simulink model "SystemPIDClosedLoop_motor_closed_zrate_cascade"  (Simulink 8.3)
settings: Solver=ode4  StartTime=0.0  StopTime=100  FixedStep=0.001  RelTol=1e-3
values from neighbouring files (symbols this model uses):
  controller = [12;  38; 4]    [layer_values.m]    (also in learnonline.m = in(end-10:end-8); learnonline1.m = in(end-10:end-8); learnonline_trial.m = in(end-10:end-8))
  delta = ones(1,4)    [ROC.m]    (also in learnonline1.m = in(end-42-((4+1)*12+(12+1)*12+(12+1)*1):end-43))
  nn_params = [Theta1(:) ; Theta2(:); Theta3(:); Theta1(:) ; Theta2(:); Theta3(:)]    [checkNNGradients.m]    (also in controller_ANN.m = in(17:end-3); jkhsgdk.m = ones(3999,1); layer_values.m = [Theta1(:); Theta2(:); Theta3(:); Theta4(:); Theta5(:); Thet; learnonline.m = [Thetap1(:); Thetap2(:); Thetap3(:); Thetac1(:); Thetac2(:);)
  plant = [14; 44; 4]    [layer_values.m]    (also in learnonline.m = in(end-13 :end-11); learnonline1.m = in(end-13 :end-11); learnonline_trial.m = in(end-13 :end-11))
undefined symbols (not defined in the file or in its folder): sumy
libraries: simulink x6, aerolibfltsims x1
settings Model: Creator=Rakhi  LastModifiedBy=binabakshi
settings SolverCC: PositivePriorityOrder=on
settings OptimizationCC: ExpressionDepthLimit=2147483647
settings DebuggingCC: FcnCallInpInsideContextMsg=UseLocalSettings
settings HardwareCC: TargetBitPerLong=64  TargetBitPerPointer=64  TargetLongLongMode=on  TargetIntDivRoundTo=Zero  TargetEndianess=LittleEndian  TargetWordSize=64  TargetHWDeviceType=MATLAB Host  ProdEqTarget=off
settings RTWCC: ProcessScript=grt_make_rtw_hook
settings GRTTargetCC: CombineOutputUpdateFcns=on  GRTInterface=off
settings ConfigurationSet: Description=SimMechanics 2G

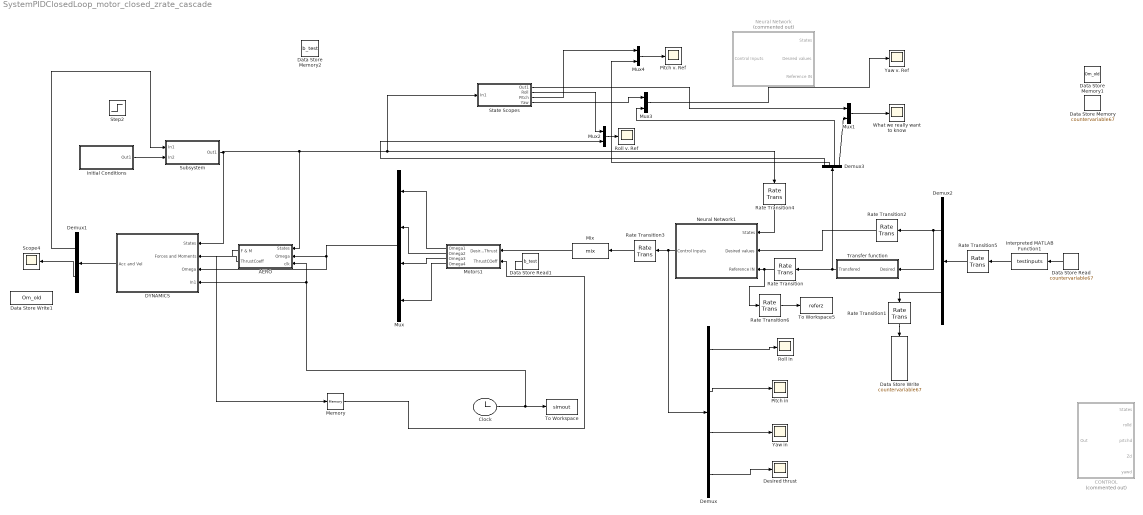
== system SystemPIDClosedLoop_motor_closed_zrate_cascade ==
  AERO : Subsystem
  CONTROL : Subsystem  Commented=on
      settings: AttributesFormatString=%<Priority>
  Clock : Clock
  DYNAMICS : Subsystem
  Data Store Memory : DataStoreMemory  DataStoreName=countervariable67
  Data Store Memory1 : DataStoreMemory  DataStoreName=Om_old  ReadBeforeWriteMsg=warning  WriteAfterWriteMsg=warning  WriteAfterReadMsg=warning
  Data Store Memory2 : DataStoreMemory  DataStoreName=b_test  ReadBeforeWriteMsg=warning  WriteAfterWriteMsg=warning  WriteAfterReadMsg=warning  InitialValue=0.000031752
  Data Store Read : DataStoreRead  DataStoreName=countervariable67  SampleTime=0.01  DataStoreElements=countervariable67
  Data Store Read1 : DataStoreRead  DataStoreName=b_test  DataStoreElements=b_test
  Data Store Write : DataStoreWrite  DataStoreName=countervariable67  DataStoreElements=countervariable67
  Data Store Write1 : DataStoreWrite  DataStoreName=Om_old  DataStoreElements=Om_old
  Demux : Demux
  Demux1 : Demux  Outputs=[12 1]
  Demux2 : Demux  Outputs=[4 1]
  Demux3 : Demux  Outputs=[1 1 1 1]
  Desired thrust : Scope
      settings: YMin=4  YMax=12  SaveName=ScopeData3
  Initial Conditions : Subsystem
  Interpreted MATLAB Function1 : MATLABFcn  MATLABFcn=testinputs  OutputDimensions=5
  Memory : Memory  X0=3.1751e-5  InheritSampleTime=on
  Mix : MATLABFcn  MATLABFcn=mix  OutputDimensions=4
  Motors1 : Subsystem
  Mux : Mux
  Mux{1..4} (4 alike) : Mux  Inputs=2
  Neural Network : Subsystem  Commented=on
  Neural Network1 : Subsystem
  Pitch in : Scope
      settings: YMin=-0.004  YMax=0.005  SaveName=ScopeData2
  Pitch v. Ref : Scope
      settings: YMin=0  YMax=0.3  SaveName=ScopeData38
  Rate Transition{,1..2,4} (4 alike) : RateTransition  OutPortSampleTime=0.01
  Rate Transition3 : RateTransition  OutPortSampleTime=0.001
  Rate Transition5 : RateTransition  OutPortSampleTime=0.001
  Rate Transition6 : RateTransition  OutPortSampleTime=0.1
  Roll in : Scope
      settings: YMin=-0.005  YMax=0.005
  Roll v. Ref : Scope
      settings: YMin=-0.2  YMax=0.5  SaveName=ScopeData35
  Scope4 : Scope
      settings: SaveName=ScopeData4
  State Scopes : Subsystem
  Subsystem : Subsystem
  To Workspace : ToWorkspace  VariableName=simout  SaveFormat=Structure  SampleTime=-1
      settings: MaxDataPoints=1
  To Workspace5 : ToWorkspace  VariableName=referz  SaveFormat=Timeseries  SampleTime=-1
      settings: MaxDataPoints=10000
  Transfer function : Subsystem
  "What we really want to know " : Scope
      settings: YMin=-3.25  YMax=0  SaveName=ScopeData32
  Yaw in : Scope
      settings: YMin=-0.45  YMax=0.5
  Yaw v. Ref : Scope
      settings: TimeRange=100  YMin=-1.5  YMax=5.5  SaveName=ScopeData37
  Step2 : Step  IOType=siggen  SampleTime=0
  wires:
  AERO/1(F & M) -> DYNAMICS/2(Forces and Moments)
  Initial Conditions/1(Out1) -> Subsystem/2(In2)
  Subsystem/1(Out1) -> DYNAMICS/1(States), AERO/1(States), Rate Transition4/1, State Scopes/1(In1)
  Demux/1 -> Roll in/1
  Demux/2 -> Pitch in/1
  Demux/4 -> Desired thrust/1
  Demux1/1 -> Subsystem/1(In1)
  DYNAMICS/1(Acc and Vel) -> Demux1/1
  Demux1/2 -> Scope4/1
  Clock/1 -> To Workspace/1, DYNAMICS/4(In1), AERO/3(clk)
  Demux/3 -> Yaw in/1
  AERO/2(ThrustCoeff) -> Memory/1
  Mix/1 -> Motors1/1(DesiredThrust)
  Data Store Read/1 -> Interpreted MATLAB Function1/1
  Mux/1 -> DYNAMICS/3(Omega), AERO/2(Omega)
  Motors1/1(Omega1) -> Mux/1
  Motors1/2(Omega2) -> Mux/2
  Motors1/3(Omega3) -> Mux/3
  Motors1/4(Omega4) -> Mux/4
  Demux2/2 -> Rate Transition1/1
  Interpreted MATLAB Function1/1 -> Rate Transition5/1
  Rate Transition1/1 -> Data Store Write/1
  Transfer function/1(Transfered) -> Rate Transition/1, Demux3/1
  Neural Network1/1(Control Inputs) -> Rate Transition3/1, Demux/1
  Demux2/1 -> Transfer function/1(Desired), Rate Transition2/1
  Rate Transition4/1 -> Neural Network1/1(States)
  Rate Transition5/1 -> Demux2/1
  Rate Transition2/1 -> Neural Network1/2(Desired values)
  Rate Transition3/1 -> Mix/1
  Rate Transition/1 -> Rate Transition6/1, Neural Network1/3(Reference IN)
  State Scopes/1(Out1) -> Mux1/1
  Mux1/1 -> "What we really want to know "/1
  Demux3/4 -> Mux1/2
  Memory/1 -> Motors1/2(ThrustCOeff)
  Rate Transition6/1 -> To Workspace5/1
  State Scopes/2("Roll ") -> Mux2/1
  Demux3/1 -> Mux2/2
  Mux2/1 -> Roll v. Ref/1
  Data Store Read1/1 -> ?
  Demux3/2 -> Mux4/2
  State Scopes/3(Pitch) -> Mux4/1
  Mux4/1 -> Pitch v. Ref/1
  Mux3/1 -> Yaw v. Ref/1
  State Scopes/4(Yaw) -> Mux3/1
  Demux3/3 -> Mux3/2

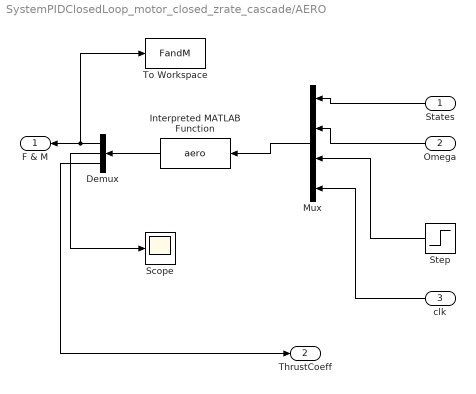
== system SystemPIDClosedLoop_motor_closed_zrate_cascade/AERO ==
  States : Inport
  Omega : Inport  Port=2
  clk : Inport  Port=3
  Demux : Demux  Outputs=[24 1 1]
  Interpreted MATLAB Function : MATLABFcn  MATLABFcn=aero
  Mux : Mux
  Scope : Scope
      settings: YMin=4.25e-07  YMax=7.75e-07  SaveName=ScopeData5
  Step : Step  Time=0  Before=4  After=4  SampleTime=0
  To Workspace : ToWorkspace  VariableName=FandM  SaveFormat=Structure  SampleTime=-1
  F & M : Outport
  ThrustCoeff : Outport  Port=2
  wires:
  Step/1 -> Mux/3
  Omega/1 -> Mux/2
  States/1 -> Mux/1
  Mux/1 -> Interpreted MATLAB Function/1
  clk/1 -> Mux/4
  Interpreted MATLAB Function/1 -> Demux/1
  Demux/1 -> F & M/1, To Workspace/1
  Demux/2 -> Scope/1
  Demux/3 -> ThrustCoeff/1

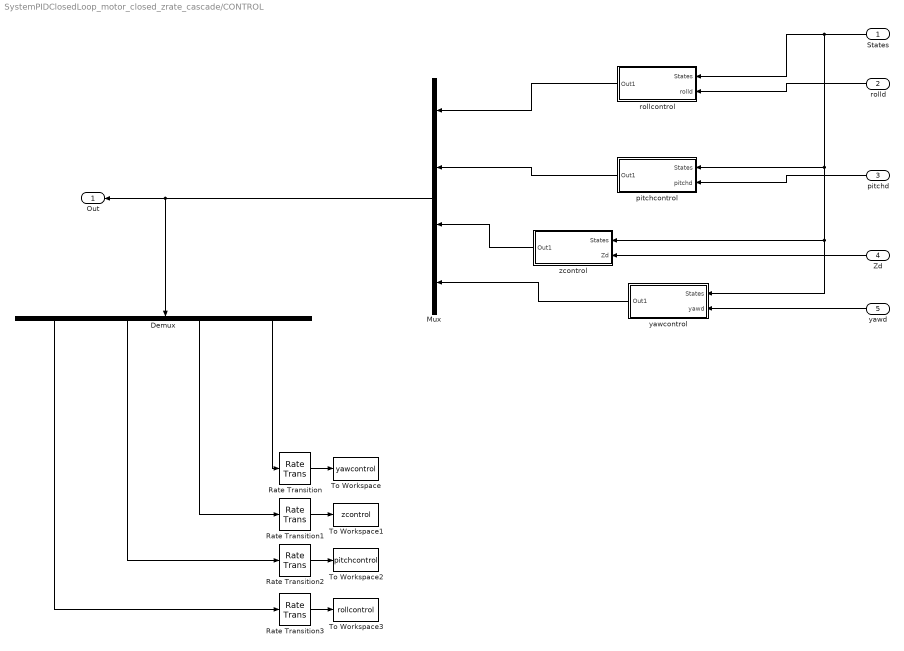
== system SystemPIDClosedLoop_motor_closed_zrate_cascade/CONTROL ==
  States : Inport
  rolld : Inport  Port=2
  pitchd : Inport  Port=3
  Zd : Inport  Port=4
  yawd : Inport  Port=5
  Demux : Demux
  Mux : Mux
  Rate Transition{,1..3} (4 alike) : RateTransition  OutPortSampleTime=0.1
  To Workspace : ToWorkspace  VariableName=yawcontrol  SaveFormat=Timeseries  SampleTime=-1
      settings: MaxDataPoints=10000  Save2DSignal=2-D array (concatenate along first dimension)
  To Workspace1 : ToWorkspace  VariableName=zcontrol  SaveFormat=Timeseries  SampleTime=-1
      settings: MaxDataPoints=10000
  To Workspace2 : ToWorkspace  VariableName=pitchcontrol  SaveFormat=Timeseries  SampleTime=-1
      settings: MaxDataPoints=10000
  To Workspace3 : ToWorkspace  VariableName=rollcontrol  SaveFormat=Timeseries  SampleTime=-1
      settings: MaxDataPoints=10000
  pitchcontrol : Subsystem
  rollcontrol : Subsystem
  yawcontrol : Subsystem
  zcontrol : Subsystem
  Out : Outport
  wires:
  States/1 -> rollcontrol/1(States), pitchcontrol/1(States), yawcontrol/1(States), zcontrol/1(States)
  rolld/1 -> rollcontrol/2(rolld)
  pitchd/1 -> pitchcontrol/2(pitchd)
  yawd/1 -> yawcontrol/2(yawd)
  Zd/1 -> zcontrol/2(Zd)
  rollcontrol/1(Out1) -> Mux/1
  pitchcontrol/1(Out1) -> Mux/2
  zcontrol/1(Out1) -> Mux/3
  yawcontrol/1(Out1) -> Mux/4
  Mux/1 -> Demux/1, Out/1
  Rate Transition1/1 -> To Workspace1/1
  Rate Transition2/1 -> To Workspace2/1
  Rate Transition3/1 -> To Workspace3/1
  Rate Transition/1 -> To Workspace/1
  Demux/4 -> Rate Transition/1
  Demux/3 -> Rate Transition1/1
  Demux/2 -> Rate Transition2/1
  Demux/1 -> Rate Transition3/1

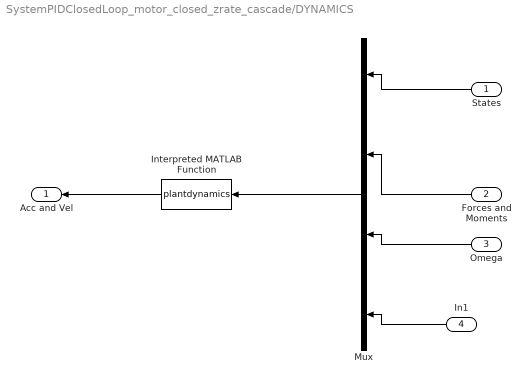
== system SystemPIDClosedLoop_motor_closed_zrate_cascade/DYNAMICS ==
  States : Inport
  Forces and Moments : Inport  Port=2
  Omega : Inport  Port=3
  In1 : Inport  Port=4
  Interpreted MATLAB Function : MATLABFcn  MATLABFcn=plantdynamics  OutputDimensions=13
  Mux : Mux
  Acc and Vel : Outport
  wires:
  States/1 -> Mux/1
  Forces and Moments/1 -> Mux/2
  Omega/1 -> Mux/3
  Mux/1 -> Interpreted MATLAB Function/1
  Interpreted MATLAB Function/1 -> Acc and Vel/1
  In1/1 -> Mux/4

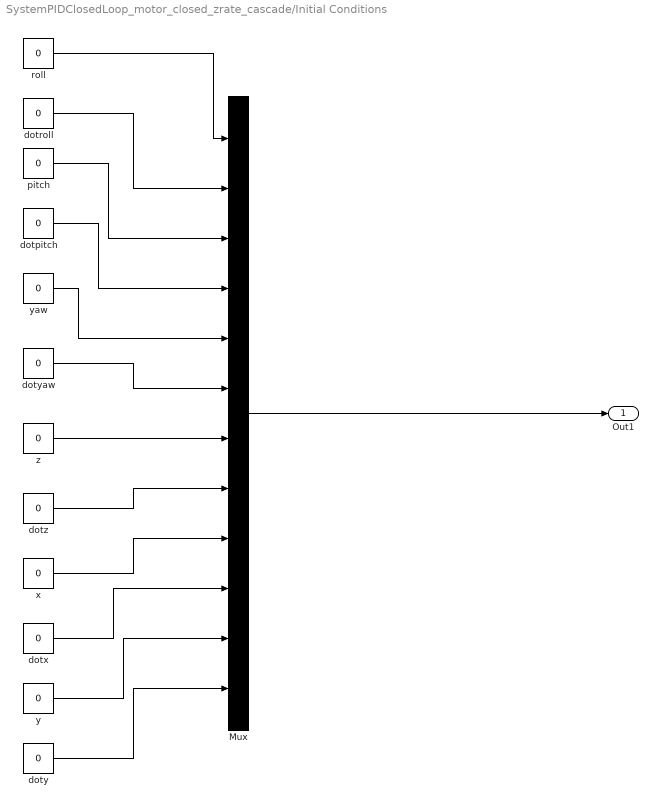
== system SystemPIDClosedLoop_motor_closed_zrate_cascade/Initial Conditions ==
  Mux : Mux  Inputs=12
  dotpitch : Constant  Value=0
  dotroll : Constant  Value=0
  dotx : Constant  Value=0
  doty : Constant  Value=0
  dotyaw : Constant  Value=0
  dotz : Constant  Value=0
  pitch : Constant  Value=0
  roll : Constant  Value=0
  x : Constant  Value=0
  y : Constant  Value=0
  yaw : Constant  Value=0
  z : Constant  Value=0
  Out1 : Outport
  wires:
  doty/1 -> Mux/12
  y/1 -> Mux/11
  dotx/1 -> Mux/10
  x/1 -> Mux/9
  dotz/1 -> Mux/8
  z/1 -> Mux/7
  dotyaw/1 -> Mux/6
  yaw/1 -> Mux/5
  dotpitch/1 -> Mux/4
  pitch/1 -> Mux/3
  dotroll/1 -> Mux/2
  roll/1 -> Mux/1
  Mux/1 -> Out1/1

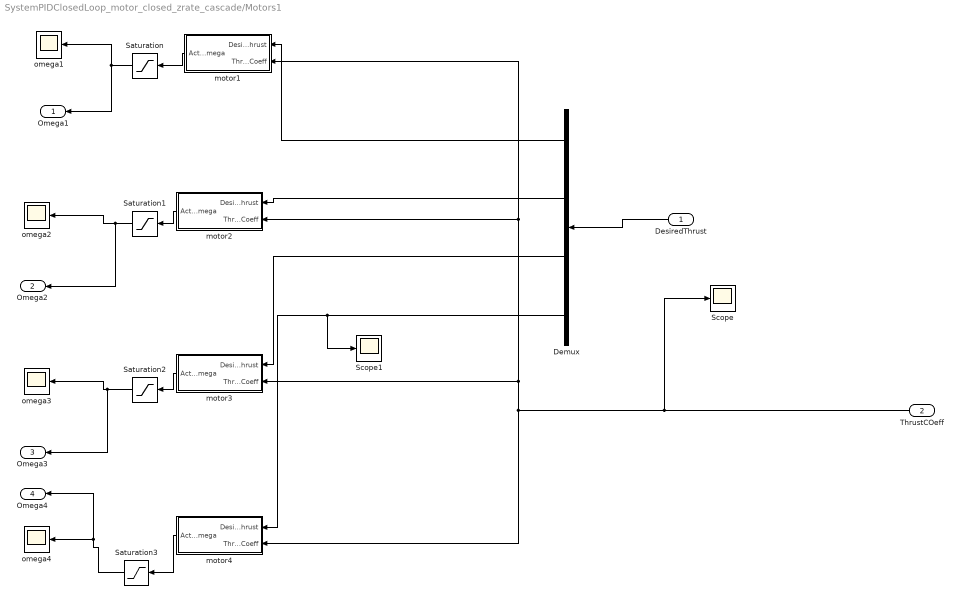
== system SystemPIDClosedLoop_motor_closed_zrate_cascade/Motors1 ==
  DesiredThrust : Inport
  ThrustCOeff : Inport  Port=2
  Demux : Demux
  Saturation{,1..3} (4 alike) : Saturate  UpperLimit=500  LowerLimit=0
  Scope : Scope
      settings: YMin=1e-05  YMax=0.00015  SaveName=ScopeData7
  Scope1 : Scope
      settings: SaveName=ScopeData26
  motor1 : Subsystem
  motor2 : Subsystem
  motor3 : Subsystem
  motor4 : Subsystem
  omega{1..4} (4 alike) : Scope
      omega1 settings: YMin=0  YMax=325  SaveName=ScopeData9
      omega2 settings: YMin=0  YMax=450  SaveName=ScopeData11
      omega3 settings: YMin=0  YMax=450  SaveName=ScopeData18
      omega4 settings: YMin=0  YMax=450  SaveName=ScopeData20
  Omega1 : Outport
  Omega2 : Outport  Port=2
  Omega3 : Outport  Port=3
  Omega4 : Outport  Port=4
  wires:
  DesiredThrust/1 -> Demux/1
  motor1/1(Actual Omega) -> Saturation/1
  motor2/1(Actual Omega) -> Saturation1/1
  motor3/1(Actual Omega) -> Saturation2/1
  motor4/1(Actual Omega) -> Saturation3/1
  Demux/1 -> motor1/1(DesiredThrust)
  ThrustCOeff/1 -> motor1/2(ThrustCoeff), motor2/2(ThrustCoeff), motor3/2(ThrustCoeff), motor4/2(ThrustCoeff), Scope/1
  Demux/2 -> motor2/1(DesiredThrust)
  Demux/3 -> motor3/1(DesiredThrust)
  Demux/4 -> motor4/1(DesiredThrust), Scope1/1
  Saturation/1 -> Omega1/1, omega1/1
  Saturation1/1 -> omega2/1, Omega2/1
  Saturation2/1 -> omega3/1, Omega3/1
  Saturation3/1 -> omega4/1, Omega4/1

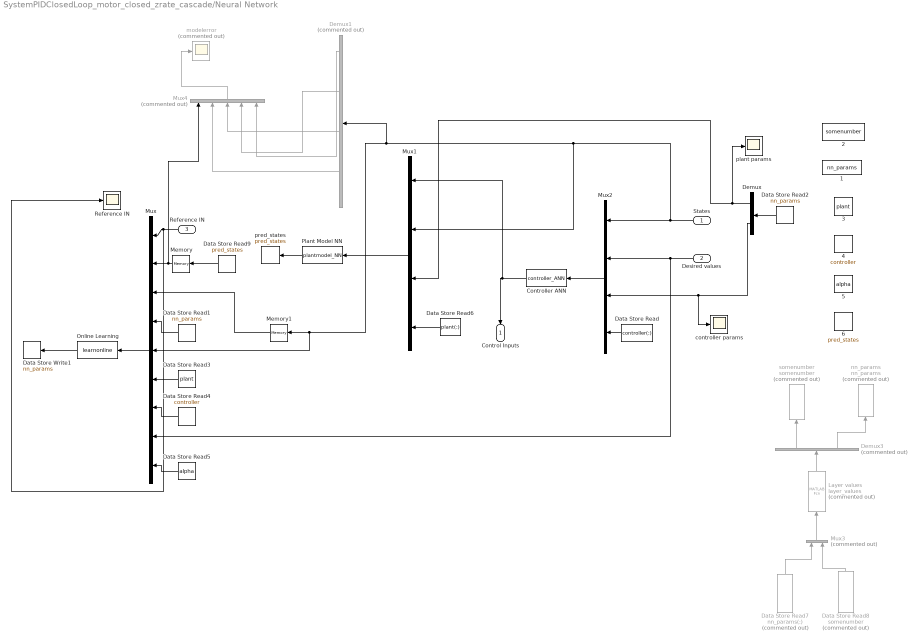
== system SystemPIDClosedLoop_motor_closed_zrate_cascade/Neural Network ==
  States : Inport
  Desired values : Inport  Port=2
  Reference IN : Inport  Port=3
  "1 " : DataStoreMemory  DataStoreName=nn_params  ReadBeforeWriteMsg=warning  WriteAfterWriteMsg=warning  WriteAfterReadMsg=warning  InitialValue=ones((14+1)*44+(44+1)*44+(44+1)*4+((12+1)*38+(38+1)*38+(38+1)*4),1)
  "2 " : DataStoreMemory  DataStoreName=somenumber  ReadBeforeWriteMsg=warning  WriteAfterWriteMsg=warning  WriteAfterReadMsg=warning
  "3 " : DataStoreMemory  DataStoreName=plant  ReadBeforeWriteMsg=warning  WriteAfterWriteMsg=warning  WriteAfterReadMsg=warning  InitialValue=[14 44 4]
  "4 " : DataStoreMemory  DataStoreName=controller  ReadBeforeWriteMsg=warning  WriteAfterWriteMsg=warning  WriteAfterReadMsg=warning  InitialValue=[12 38 4]
  "5 " : DataStoreMemory  DataStoreName=alpha  ReadBeforeWriteMsg=warning  WriteAfterWriteMsg=warning  WriteAfterReadMsg=warning  InitialValue=[0.001 0.01 0.1 0.1]
  "6 " : DataStoreMemory  DataStoreName=pred_states  ReadBeforeWriteMsg=warning  WriteAfterWriteMsg=warning  WriteAfterReadMsg=warning  InitialValue=[0;0;0;0]
  Controller ANN : MATLABFcn  MATLABFcn=controller_ANN
  Data Store Read : DataStoreRead  DataStoreName=controller  SampleTime=0.001  DataStoreElements=controller(:)
  Data Store Read1 : DataStoreRead  DataStoreName=nn_params  SampleTime=0.001  DataStoreElements=nn_params
  Data Store Read2 : DataStoreRead  DataStoreName=nn_params  SampleTime=0.001  DataStoreElements=nn_params
  Data Store Read3 : DataStoreRead  DataStoreName=plant  SampleTime=0.001  DataStoreElements=plant
  Data Store Read4 : DataStoreRead  DataStoreName=controller  SampleTime=0.001  DataStoreElements=controller
  Data Store Read5 : DataStoreRead  DataStoreName=alpha  SampleTime=0.001  DataStoreElements=alpha
  Data Store Read6 : DataStoreRead  DataStoreName=plant  SampleTime=0.001  DataStoreElements=plant(:)
  Data Store Read7 : DataStoreRead  Commented=on  DataStoreName=nn_params  DataStoreElements=nn_params(:)
  Data Store Read8 : DataStoreRead  Commented=on  DataStoreName=somenumber  DataStoreElements=somenumber
  Data Store Read9 : DataStoreRead  DataStoreName=pred_states  SampleTime=0.001  DataStoreElements=pred_states
  Data Store Write1 : DataStoreWrite  DataStoreName=nn_params  DataStoreElements=nn_params
  Demux : Demux  Outputs=[((14+1)*44+(44+1)*44+(44+1)*4) ((12+1)*38+(38+1)*38+(38+1)*4)]
  Demux1 : Demux  Commented=on  Outputs=[1 1 1 1 1 1 1 5]
  Demux3 : Demux  Commented=on  Outputs=[1 ((14+1)*44+(44+1)*44+(44+1)*4)+((12+1)*38+(38+1)*38+(38+1)*4)]
  Layer values : MATLABFcn  Commented=on  MATLABFcn=layer_values
  Memory : Memory
  Memory1 : Memory
  Mux : Mux  Inputs=9
  Mux1 : Mux  Inputs=[4 12 2820 3]
  Mux2 : Mux  Inputs=[12 4 2132 3]
  Mux3 : Mux  Commented=on  Inputs=2
  Mux4 : Mux  Commented=on  Inputs=[4 1 1 1 1]
  Online Learning : MATLABFcn  MATLABFcn=learnonline
  Plant Model NN : MATLABFcn  MATLABFcn=plantmodel_NN
  "Reference IN " : Scope
      settings: YMin=-0.35  YMax=0  SaveName=ScopeData22
  "controller params " : Scope
      settings: YMin=-12.5  YMax=7.5  SaveName=ScopeData23
  "modelerror " : Scope  Commented=on
      settings: YMin=0  YMax=35  SaveName=ScopeData21
  nn_params : DataStoreWrite  Commented=on  DataStoreName=nn_params  DataStoreElements=nn_params
  "plant params " : Scope
      settings: YMin=-1.75  YMax=3  SaveName=ScopeData28
  pred_states : DataStoreWrite  DataStoreName=pred_states  DataStoreElements=pred_states
  somenumber : DataStoreWrite  Commented=on  DataStoreName=somenumber  DataStoreElements=somenumber
  Control Inputs : Outport
  wires:
  Mux2/1 -> Controller ANN/1
  Desired values/1 -> Mux/8, Mux2/2
  Mux1/1 -> Plant Model NN/1
  Controller ANN/1 -> Mux1/1, Control Inputs/1
  Mux/1 -> Online Learning/1
  Reference IN/1 -> "Reference IN "/1, Mux/1
  Demux3/1 -> somenumber/1
  Demux3/2 -> nn_params/1
  Demux/2 -> "controller params "/1, Mux2/3
  Data Store Read1/1 -> Mux/4
  Data Store Read3/1 -> Mux/6
  Data Store Read4/1 -> Mux/7
  Data Store Read5/1 -> Mux/9
  Data Store Read6/1 -> Mux1/4
  Data Store Read/1 -> Mux2/4
  Demux/1 -> "plant params "/1, Mux1/3
  Layer values/1 -> Demux3/1
  Data Store Read8/1 -> Mux3/2
  Data Store Read2/1 -> Demux/1
  Data Store Read7/1 -> Mux3/1
  Mux3/1 -> Layer values/1
  Mux4/1 -> "modelerror "/1
  Plant Model NN/1 -> pred_states/1
  States/1 -> Mux1/2, Demux1/1, Mux/5, Memory1/1, Mux2/1
  Demux1/1 -> Mux4/5
  Demux1/3 -> Mux4/4
  Demux1/5 -> Mux4/3
  Demux1/7 -> Mux4/2
  Online Learning/1 -> Data Store Write1/1
  Data Store Read9/1 -> Memory/1
  Memory/1 -> Mux4/1, Mux/2
  Memory1/1 -> Mux/3

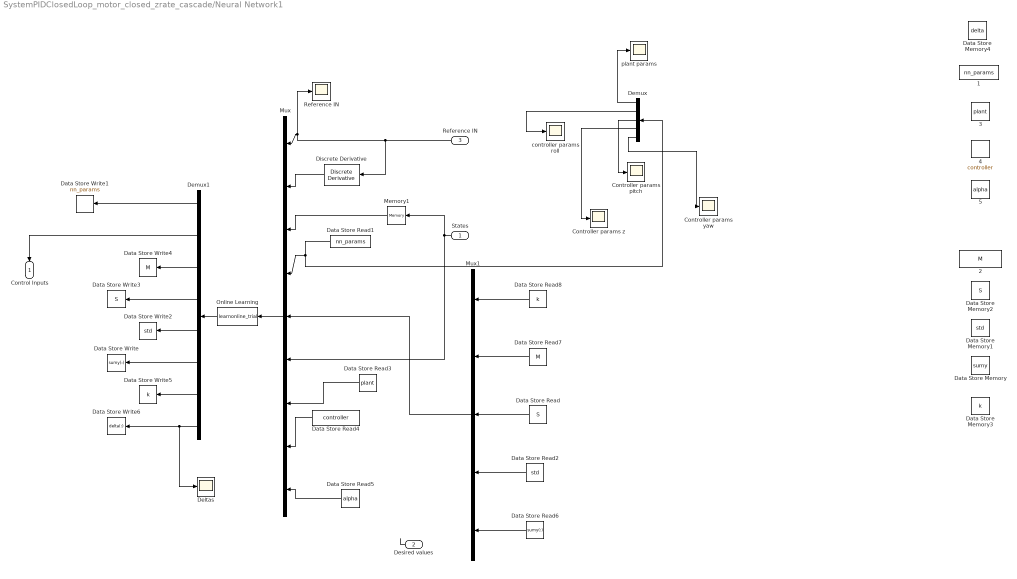
== system SystemPIDClosedLoop_motor_closed_zrate_cascade/Neural Network1 ==
  States : Inport
  Desired values : Inport  Port=2
  Reference IN : Inport  Port=3
  "1 " : DataStoreMemory  DataStoreName=nn_params  ReadBeforeWriteMsg=warning  WriteAfterWriteMsg=warning  WriteAfterReadMsg=warning  InitialValue=ones((14+1)*44+(44+1)*44+(44+1)*4+20,1)
  "2 " : DataStoreMemory  DataStoreName=M  ReadBeforeWriteMsg=warning  WriteAfterWriteMsg=warning  WriteAfterReadMsg=warning  InitialValue=zeros(16,1)
  "3 " : DataStoreMemory  DataStoreName=plant  ReadBeforeWriteMsg=warning  WriteAfterWriteMsg=warning  WriteAfterReadMsg=warning  InitialValue=[14 44 4]
  "4 " : DataStoreMemory  DataStoreName=controller  ReadBeforeWriteMsg=warning  WriteAfterWriteMsg=warning  WriteAfterReadMsg=warning  InitialValue=[4 12 1]
  "5 " : DataStoreMemory  DataStoreName=alpha  ReadBeforeWriteMsg=warning  WriteAfterWriteMsg=warning  WriteAfterReadMsg=warning  InitialValue=[0.01 0.01 0.01 0.001 10 0 0 0]
  "Controller params pitch " : Scope
      settings: YMin=-1.2  YMax=1  SaveName=ScopeData30
  Controller params yaw : Scope
      settings: YMin=-0.75  YMax=2.5  SaveName=ScopeData34
  Controller params z : Scope
      settings: YMin=-1.5  YMax=5.5  SaveName=ScopeData31
  Data Store Memory : DataStoreMemory  DataStoreName=sumy  ReadBeforeWriteMsg=warning  WriteAfterWriteMsg=warning  WriteAfterReadMsg=warning  InitialValue=zeros(16,1)
  Data Store Memory1 : DataStoreMemory  DataStoreName=std  ReadBeforeWriteMsg=warning  WriteAfterWriteMsg=warning  WriteAfterReadMsg=warning  InitialValue=zeros(16,1)
  Data Store Memory2 : DataStoreMemory  DataStoreName=S  ReadBeforeWriteMsg=warning  WriteAfterWriteMsg=warning  WriteAfterReadMsg=warning  InitialValue=zeros(16,1)
  Data Store Memory3 : DataStoreMemory  DataStoreName=k  ReadBeforeWriteMsg=warning  WriteAfterWriteMsg=warning  WriteAfterReadMsg=warning  Dimensions=1
  Data Store Memory4 : DataStoreMemory  DataStoreName=delta  ReadBeforeWriteMsg=warning  WriteAfterWriteMsg=warning  WriteAfterReadMsg=warning  InitialValue=ones(20,1)
  Data Store Read : DataStoreRead  DataStoreName=S  DataStoreElements=S
  Data Store Read1 : DataStoreRead  DataStoreName=nn_params  SampleTime=0.01  DataStoreElements=nn_params
  Data Store Read2 : DataStoreRead  DataStoreName=std  DataStoreElements=std
  Data Store Read3 : DataStoreRead  DataStoreName=plant  SampleTime=0.01  DataStoreElements=plant
  Data Store Read4 : DataStoreRead  DataStoreName=controller  SampleTime=0.01  DataStoreElements=controller
  Data Store Read5 : DataStoreRead  DataStoreName=alpha  SampleTime=0.01  DataStoreElements=alpha
  Data Store Read6 : DataStoreRead  DataStoreName=sumy  DataStoreElements=sumy(:)
  Data Store Read7 : DataStoreRead  DataStoreName=M  DataStoreElements=M
  Data Store Read8 : DataStoreRead  DataStoreName=k  DataStoreElements=k
  Data Store Write : DataStoreWrite  DataStoreName=sumy  DataStoreElements=sumy(:)
  Data Store Write1 : DataStoreWrite  DataStoreName=nn_params  DataStoreElements=nn_params
  Data Store Write2 : DataStoreWrite  DataStoreName=std  DataStoreElements=std
  Data Store Write3 : DataStoreWrite  DataStoreName=S  DataStoreElements=S
  Data Store Write4 : DataStoreWrite  DataStoreName=M  DataStoreElements=M
  Data Store Write5 : DataStoreWrite  DataStoreName=k  DataStoreElements=k
  Data Store Write6 : DataStoreWrite  DataStoreName=delta  DataStoreElements=delta(:)
  "Deltas " : Scope
      settings: YMin=-32.5  YMax=15  SaveName=ScopeData33
  Demux : Demux  Outputs=[((14+1)*44+(44+1)*44+(44+1)*4) 5 5 5 5]
  Demux1 : Demux  Outputs=[((14+1)*44+(44+1)*44+(44+1)*4+20) 4 16 16 16 16 1 20]
  Discrete Derivative : simulink/Discrete/Discrete Derivative  gainval=1.0  ICPrevScaledInput=0.0  InputProcessing=Inherited  OutMin=[]  OutMax=[]  OutDataType=fixdt(1, 16)  OutScaling=2^-10  DoSatur=off
  Memory1 : Memory  InheritSampleTime=on
  Mux : Mux  Inputs=9
  Mux1 : Mux  Inputs=5
  Online Learning : MATLABFcn  MATLABFcn=learnonline_trial
  "Reference IN " : Scope
      settings: YMin=-11  YMax=0  SaveName=ScopeData22
  "controller params roll   " : Scope
      settings: YMin=-1.1  YMax=1  SaveName=ScopeData23
  "plant params " : Scope
      settings: TimeRange=10  YMin=-2  YMax=1.5  SaveName=ScopeData28
  Control Inputs : Outport
  wires:
  Desired values/1 -> ?
  Demux1/2 -> Control Inputs/1
  Mux/1 -> Online Learning/1
  Reference IN/1 -> Discrete Derivative/1, "Reference IN "/1, Mux/1
  Demux/2 -> "controller params roll   "/1
  Data Store Read3/1 -> Mux/7
  Data Store Read4/1 -> Mux/8
  Demux/1 -> "plant params "/1
  Data Store Read1/1 -> Mux/4, Demux/1
  States/1 -> Mux/6, Memory1/1
  Demux1/1 -> Data Store Write1/1
  Discrete Derivative/1 -> Mux/2
  Memory1/1 -> Mux/3
  Online Learning/1 -> Demux1/1
  Demux/3 -> "Controller params pitch "/1
  Demux/4 -> Controller params z/1
  Demux1/6 -> Data Store Write/1
  Demux1/5 -> Data Store Write2/1
  Demux1/4 -> Data Store Write3/1
  Demux1/3 -> Data Store Write4/1
  Demux1/7 -> Data Store Write5/1
  Data Store Read7/1 -> Mux1/2
  Data Store Read6/1 -> Mux1/5
  Data Store Read2/1 -> Mux1/4
  Data Store Read/1 -> Mux1/3
  Data Store Read8/1 -> Mux1/1
  Mux1/1 -> Mux/5
  Demux1/8 -> "Deltas "/1, Data Store Write6/1
  Data Store Read5/1 -> Mux/9
  Demux/5 -> Controller params yaw/1

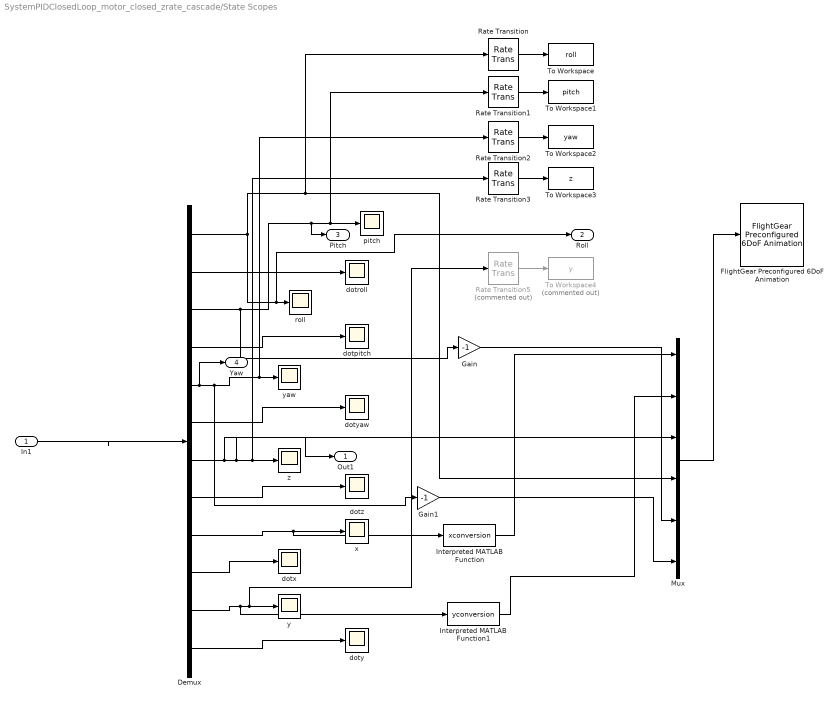
== system SystemPIDClosedLoop_motor_closed_zrate_cascade/State Scopes ==
  In1 : Inport
  Demux : Demux  Outputs=12
  FlightGear Preconfigured 6DoF Animation : aerolibfltsims/FlightGear Preconfigured 6DoF Animation  xFlightGearVersion=v2.12  DestinationIpAddress=127.0.0.1  DestinationPort=5502  SampleTime=-1
  Gain : Gain  Gain=-1
  Gain1 : Gain  Gain=-1
  Interpreted MATLAB Function : MATLABFcn  MATLABFcn=xconversion
  Interpreted MATLAB Function1 : MATLABFcn  MATLABFcn=yconversion
  Mux : Mux  Inputs=6
  Rate Transition{,1..3} (4 alike) : RateTransition  OutPortSampleTime=0.1
  Rate Transition5 : RateTransition  Commented=on  OutPortSampleTime=0.1
  To Workspace : ToWorkspace  VariableName=roll  SaveFormat=Timeseries  SampleTime=-1
      settings: MaxDataPoints=10000  Save2DSignal=2-D array (concatenate along first dimension)
  To Workspace1 : ToWorkspace  VariableName=pitch  SaveFormat=Timeseries  SampleTime=-1
      settings: MaxDataPoints=10000
  To Workspace2 : ToWorkspace  VariableName=yaw  SaveFormat=Timeseries  SampleTime=-1
      settings: MaxDataPoints=10000
  To Workspace3 : ToWorkspace  VariableName=z  SaveFormat=Timeseries  SampleTime=-1
      settings: MaxDataPoints=10000
  To Workspace4 : ToWorkspace  Commented=on  VariableName=y  SaveFormat=Timeseries  SampleTime=-1
      settings: MaxDataPoints=10000
  dotpitch : Scope
      settings: YMin=-0.07  YMax=0.1  SaveName=ScopeData8
  dotroll : Scope
      settings: YMin=-0.35  YMax=0.35  SaveName=ScopeData6
  dotx : Scope
      settings: YMin=-4  YMax=0.25  SaveName=ScopeData14
  doty : Scope
      settings: SaveName=ScopeData16
  dotyaw : Scope
      settings: YMin=-0.175  YMax=0.275  SaveName=ScopeData10
  dotz : Scope
      settings: YMin=-1.5  YMax=1.25  SaveName=ScopeData12
  pitch : Scope
      settings: YMin=-2  YMax=1  SaveName=sc_pitch
  roll : Scope
      settings: YMin=0  YMax=1.1  SaveName=sc_roll
  x : Scope
      settings: SaveName=ScopeData13
  y : Scope
      settings: TimeRange=0.7999999999999972  YMin=2600  YMax=2780  SaveName=ScopeData15
  yaw : Scope
      settings: YMin=-50  YMax=2.5  SaveName=sc_yaw
  z : Scope
      settings: YMin=-10.6  YMax=-9.65  SaveName=sc_z
  Out1 : Outport
  "Roll " : Outport  Port=2
  Pitch : Outport  Port=3
  Yaw : Outport  Port=4
  wires:
  In1/1 -> Demux/1
  Demux/1 -> Rate Transition/1, Mux/4, "Roll "/1, roll/1
  Demux/2 -> dotroll/1
  Demux/3 -> Pitch/1, Rate Transition1/1, pitch/1, Gain/1
  Demux/4 -> dotpitch/1
  Demux/5 -> Yaw/1, Rate Transition2/1, yaw/1, Gain1/1
  Demux/6 -> dotyaw/1
  Demux/7 -> Out1/1, Mux/3, Rate Transition3/1, z/1
  Demux/8 -> dotz/1
  Demux/9 -> x/1, Interpreted MATLAB Function/1
  Demux/10 -> dotx/1
  Demux/11 -> Rate Transition5/1, y/1, Interpreted MATLAB Function1/1
  Demux/12 -> doty/1
  Interpreted MATLAB Function1/1 -> Mux/2
  Interpreted MATLAB Function/1 -> Mux/1
  Mux/1 -> FlightGear Preconfigured 6DoF Animation/1
  Gain/1 -> Mux/5
  Gain1/1 -> Mux/6
  Rate Transition1/1 -> To Workspace1/1
  Rate Transition2/1 -> To Workspace2/1
  Rate Transition3/1 -> To Workspace3/1
  Rate Transition5/1 -> To Workspace4/1
  Rate Transition/1 -> To Workspace/1

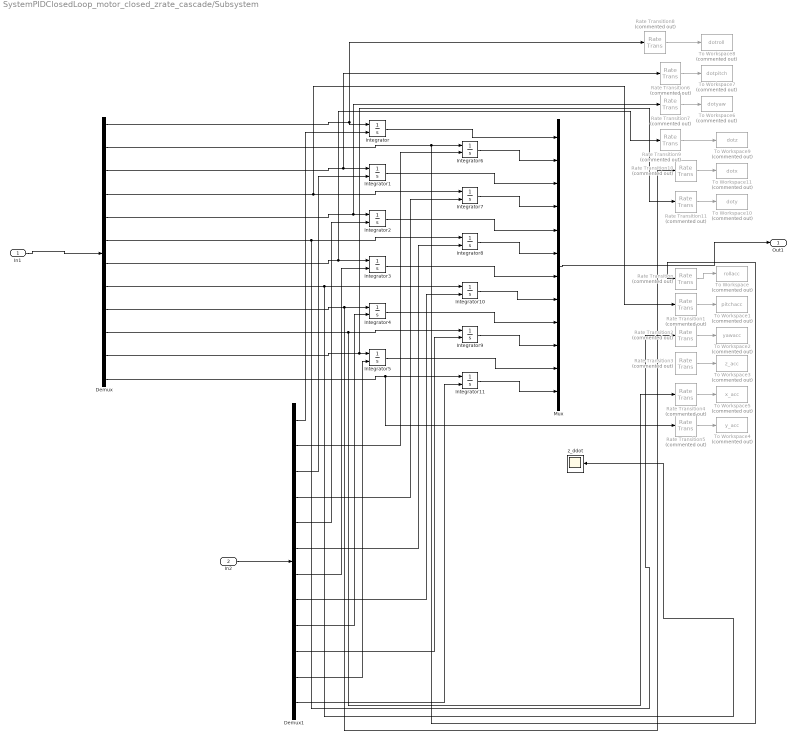
== system SystemPIDClosedLoop_motor_closed_zrate_cascade/Subsystem ==
  In1 : Inport
  In2 : Inport  Port=2
  Demux : Demux  Outputs=12
  Demux1 : Demux  Outputs=12
  Integrator{,1..11} (12 alike) : Integrator  InitialConditionSource=external
  Mux : Mux  Inputs=12
  Rate Transition{,1..11} (12 alike) : RateTransition  Commented=on  OutPortSampleTime=0.1
  To Workspace : ToWorkspace  Commented=on  VariableName=rollacc  SaveFormat=Timeseries  SampleTime=-1
      settings: MaxDataPoints=10000  Save2DSignal=2-D array (concatenate along first dimension)
  To Workspace1 : ToWorkspace  Commented=on  VariableName=pitchacc  SaveFormat=Timeseries  SampleTime=-1
      settings: MaxDataPoints=10000
  To Workspace10 : ToWorkspace  Commented=on  VariableName=doty  SaveFormat=Timeseries  SampleTime=-1
      settings: MaxDataPoints=10000
  To Workspace11 : ToWorkspace  Commented=on  VariableName=dotx  SaveFormat=Timeseries  SampleTime=-1
      settings: MaxDataPoints=10000
  To Workspace2 : ToWorkspace  Commented=on  VariableName=yawacc  SaveFormat=Timeseries  SampleTime=-1
      settings: MaxDataPoints=10000
  To Workspace3 : ToWorkspace  Commented=on  VariableName=z_acc  SaveFormat=Timeseries  SampleTime=-1
      settings: MaxDataPoints=10000
  To Workspace4 : ToWorkspace  Commented=on  VariableName=y_acc  SaveFormat=Timeseries  SampleTime=-1
      settings: MaxDataPoints=10000
  To Workspace5 : ToWorkspace  Commented=on  VariableName=x_acc  SaveFormat=Timeseries  SampleTime=-1
      settings: MaxDataPoints=10000
  To Workspace6 : ToWorkspace  Commented=on  VariableName=dotyaw  SaveFormat=Timeseries  SampleTime=-1
      settings: MaxDataPoints=10000
  To Workspace7 : ToWorkspace  Commented=on  VariableName=dotpitch  SaveFormat=Timeseries  SampleTime=-1
      settings: MaxDataPoints=10000
  To Workspace8 : ToWorkspace  Commented=on  VariableName=dotroll  SaveFormat=Timeseries  SampleTime=-1
      settings: MaxDataPoints=10000
  To Workspace9 : ToWorkspace  Commented=on  VariableName=dotz  SaveFormat=Timeseries  SampleTime=-1
      settings: MaxDataPoints=10000
  z_ddot : Scope
      settings: YMin=-3  YMax=2  SaveName=ScopeData36
  Out1 : Outport
  wires:
  Demux/1 -> Rate Transition8/1, Integrator/1
  Demux/2 -> Rate Transition/1, Integrator6/1
  Demux/3 -> Rate Transition6/1, Integrator1/1
  Demux/4 -> Rate Transition1/1, Integrator7/1
  Demux/5 -> Rate Transition7/1, Integrator2/1
  Demux/6 -> Rate Transition2/1, Integrator8/1
  Demux/7 -> Rate Transition9/1, Integrator3/1
  Demux/8 -> z_ddot/1, Integrator10/1
  Demux/9 -> Rate Transition10/1, Integrator4/1
  Demux/10 -> Rate Transition4/1, Integrator9/1
  Demux/11 -> Rate Transition11/1, Integrator5/1
  Demux/12 -> Rate Transition5/1, Integrator11/1
  In1/1 -> Demux/1
  Demux1/1 -> Integrator/2
  Demux1/2 -> Integrator6/2
  Demux1/3 -> Integrator1/2
  Demux1/4 -> Integrator7/2
  Demux1/5 -> Integrator2/2
  Demux1/6 -> Integrator8/2
  Demux1/7 -> Integrator3/2
  Demux1/8 -> Integrator10/2
  Demux1/9 -> Integrator4/2
  Demux1/10 -> Integrator9/2
  Demux1/11 -> Integrator5/2
  Demux1/12 -> Integrator11/2
  In2/1 -> Demux1/1
  Integrator/1 -> Mux/1
  Integrator6/1 -> Mux/2
  Integrator1/1 -> Mux/3
  Integrator7/1 -> Mux/4
  Integrator2/1 -> Mux/5
  Integrator8/1 -> Mux/6
  Integrator10/1 -> Mux/8
  Integrator4/1 -> Mux/9
  Integrator9/1 -> Mux/10
  Integrator5/1 -> Mux/11
  Integrator11/1 -> Mux/12
  Mux/1 -> Out1/1
  Rate Transition1/1 -> To Workspace1/1
  Rate Transition2/1 -> To Workspace2/1
  Rate Transition3/1 -> To Workspace3/1
  Rate Transition4/1 -> To Workspace5/1
  Rate Transition5/1 -> To Workspace4/1
  Rate Transition/1 -> To Workspace/1
  Rate Transition9/1 -> To Workspace9/1
  Rate Transition10/1 -> To Workspace11/1
  Rate Transition11/1 -> To Workspace10/1
  Rate Transition8/1 -> To Workspace8/1
  Rate Transition6/1 -> To Workspace7/1
  Rate Transition7/1 -> To Workspace6/1
  Integrator3/1 -> Mux/7

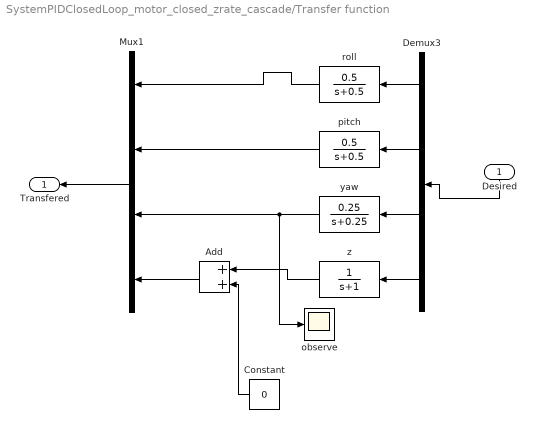
== system SystemPIDClosedLoop_motor_closed_zrate_cascade/Transfer function ==
  Desired : Inport
  Add : Sum
  Constant : Constant  Value=0
  Demux3 : Demux
  Mux1 : Mux
  "observe " : Scope
      settings: YMin=-3.5  YMax=3  SaveName=ScopeData19
  pitch : TransferFcn  Numerator=[0 0 0.5]  Denominator=[0 1 0.5]
  roll : TransferFcn  Numerator=[0 0.5]  Denominator=[1 0.5]
  yaw : TransferFcn  Numerator=[0 0 0.25]  Denominator=[0 1 0.25]
  z : TransferFcn  Numerator=[0 1]  Denominator=[1 1]
  Transfered : Outport
  wires:
  yaw/1 -> "observe "/1, Mux1/3
  Desired/1 -> Demux3/1
  Demux3/4 -> z/1
  Demux3/1 -> roll/1
  z/1 -> Add/1
  Demux3/2 -> pitch/1
  Demux3/3 -> yaw/1
  roll/1 -> Mux1/1
  Mux1/1 -> Transfered/1
  pitch/1 -> Mux1/2
  Add/1 -> Mux1/4
  Constant/1 -> Add/2

== system SystemPIDClosedLoop_motor_closed_zrate_cascade/CONTROL/pitchcontrol ==
  States : Inport
  pitchd : Inport  Port=2
  Interpreted MATLAB Function : MATLABFcn  MATLABFcn=pitcherr  OutputDimensions=1
  Mux : Mux  Inputs=2
  PID Controller : simulink/Continuous/PID Controller  Controller=PID  TimeDomain=Continuous-time  SampleTime=1  IntegratorMethod=Forward Euler  FilterMethod=Forward Euler  Form=Parallel  P=0.005  I=0  D=0.025  N=25  InitialConditionSource=internal  InitialConditionForIntegrator=0  InitialConditionForFilter=0  ExternalReset=none  LimitOutput=off  UpperSaturationLimit=inf  LowerSaturationLimit=-inf  LinearizeAsGain=off  AntiWindupMode=none  Kb=1  TrackingMode=off  Kt=1  PParamMin=[]  PParamMax=[]  IParamMin=[]  IParamMax=[]  DParamMin=[]  DParamMax=[]  NParamMin=[]  NParamMax=[]  KbParamMin=[]  KbParamMax=[]  KtParamMin=[]  KtParamMax=[]  POutMin=[]  POutMax=[]  IOutMin=[]  IOutMax=[]  DOutMin=[]  DOutMax=[]  NOutMin=[]  NOutMax=[]  KbOutMin=[]  KbOutMax=[]  KtOutMin=[]  KtOutMax=[]  IntegratorOutMin=[]  IntegratorOutMax=[]  FilterOutMin=[]  FilterOutMax=[]  SumOutMin=[]  SumOutMax=[]  SumI1OutMin=[]  SumI1OutMax=[]  SumI2OutMin=[]  SumI2OutMax=[]  SumI3OutMin=[]  SumI3OutMax=[]  SumDOutMin=[]  SumDOutMax=[]  SaturationOutMin=[]  SaturationOutMax=[]  IntegratorContinuousStateAttributes=''  IntegratorStateMustResolveToSignalObject=off  IntegratorRTWStateStorageClass=Auto  FilterContinuousStateAttributes=''  FilterStateMustResolveToSignalObject=off  FilterRTWStateStorageClass=Auto
  Out1 : Outport
  wires:
  States/1 -> Mux/1
  pitchd/1 -> Mux/2
  Mux/1 -> Interpreted MATLAB Function/1
  Interpreted MATLAB Function/1 -> PID Controller/1
  PID Controller/1 -> Out1/1

== system SystemPIDClosedLoop_motor_closed_zrate_cascade/CONTROL/rollcontrol ==
  States : Inport
  rolld : Inport  Port=2
  Interpreted MATLAB Function : MATLABFcn  MATLABFcn=rollerr  OutputDimensions=1
  Mux : Mux  Inputs=2
  PID Controller : simulink/Continuous/PID Controller  Controller=PID  TimeDomain=Continuous-time  SampleTime=1  IntegratorMethod=Forward Euler  FilterMethod=Forward Euler  Form=Parallel  P=.005  I=0  D=.025  N=25  InitialConditionSource=internal  InitialConditionForIntegrator=0  InitialConditionForFilter=0  ExternalReset=none  LimitOutput=off  UpperSaturationLimit=inf  LowerSaturationLimit=-inf  LinearizeAsGain=off  AntiWindupMode=none  Kb=1  TrackingMode=off  Kt=1  PParamMin=[]  PParamMax=[]  IParamMin=[]  IParamMax=[]  DParamMin=[]  DParamMax=[]  NParamMin=[]  NParamMax=[]  KbParamMin=[]  KbParamMax=[]  KtParamMin=[]  KtParamMax=[]  POutMin=[]  POutMax=[]  IOutMin=[]  IOutMax=[]  DOutMin=[]  DOutMax=[]  NOutMin=[]  NOutMax=[]  KbOutMin=[]  KbOutMax=[]  KtOutMin=[]  KtOutMax=[]  IntegratorOutMin=[]  IntegratorOutMax=[]  FilterOutMin=[]  FilterOutMax=[]  SumOutMin=[]  SumOutMax=[]  SumI1OutMin=[]  SumI1OutMax=[]  SumI2OutMin=[]  SumI2OutMax=[]  SumI3OutMin=[]  SumI3OutMax=[]  SumDOutMin=[]  SumDOutMax=[]  SaturationOutMin=[]  SaturationOutMax=[]  IntegratorContinuousStateAttributes=''  IntegratorStateMustResolveToSignalObject=off  IntegratorRTWStateStorageClass=Auto  FilterContinuousStateAttributes=''  FilterStateMustResolveToSignalObject=off  FilterRTWStateStorageClass=Auto
  Out1 : Outport
  wires:
  States/1 -> Mux/1
  rolld/1 -> Mux/2
  Mux/1 -> Interpreted MATLAB Function/1
  Interpreted MATLAB Function/1 -> PID Controller/1
  PID Controller/1 -> Out1/1

== system SystemPIDClosedLoop_motor_closed_zrate_cascade/CONTROL/yawcontrol ==
  States : Inport
  yawd : Inport  Port=2
  Interpreted MATLAB Function : MATLABFcn  MATLABFcn=yawerr  OutputDimensions=1
  Mux : Mux  Inputs=2
  PID Controller : simulink/Continuous/PID Controller  Controller=PID  TimeDomain=Continuous-time  SampleTime=1  IntegratorMethod=Forward Euler  FilterMethod=Forward Euler  Form=Parallel  P=0.05  I=0  D=0.25  N=25  InitialConditionSource=internal  InitialConditionForIntegrator=0  InitialConditionForFilter=0  ExternalReset=none  LimitOutput=off  UpperSaturationLimit=inf  LowerSaturationLimit=-inf  LinearizeAsGain=off  AntiWindupMode=none  Kb=1  TrackingMode=off  Kt=1  PParamMin=[]  PParamMax=[]  IParamMin=[]  IParamMax=[]  DParamMin=[]  DParamMax=[]  NParamMin=[]  NParamMax=[]  KbParamMin=[]  KbParamMax=[]  KtParamMin=[]  KtParamMax=[]  POutMin=[]  POutMax=[]  IOutMin=[]  IOutMax=[]  DOutMin=[]  DOutMax=[]  NOutMin=[]  NOutMax=[]  KbOutMin=[]  KbOutMax=[]  KtOutMin=[]  KtOutMax=[]  IntegratorOutMin=[]  IntegratorOutMax=[]  FilterOutMin=[]  FilterOutMax=[]  SumOutMin=[]  SumOutMax=[]  SumI1OutMin=[]  SumI1OutMax=[]  SumI2OutMin=[]  SumI2OutMax=[]  SumI3OutMin=[]  SumI3OutMax=[]  SumDOutMin=[]  SumDOutMax=[]  SaturationOutMin=[]  SaturationOutMax=[]  IntegratorContinuousStateAttributes=''  IntegratorStateMustResolveToSignalObject=off  IntegratorRTWStateStorageClass=Auto  FilterContinuousStateAttributes=''  FilterStateMustResolveToSignalObject=off  FilterRTWStateStorageClass=Auto
  Scope : Scope
      settings: SaveName=ScopeData17
  Out1 : Outport
  wires:
  States/1 -> Mux/1
  yawd/1 -> Mux/2
  Mux/1 -> Interpreted MATLAB Function/1
  Interpreted MATLAB Function/1 -> PID Controller/1, Scope/1
  PID Controller/1 -> Out1/1

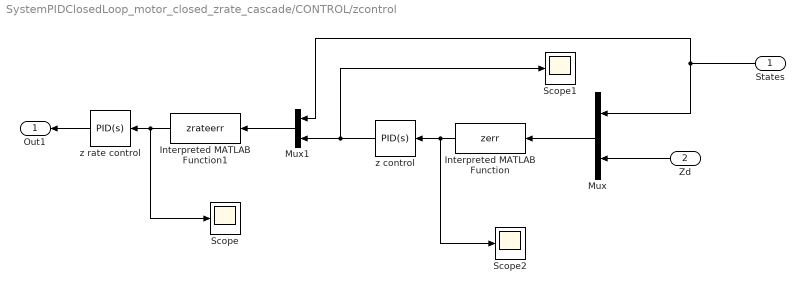
== system SystemPIDClosedLoop_motor_closed_zrate_cascade/CONTROL/zcontrol ==
  States : Inport
  Zd : Inport  Port=2
  Interpreted MATLAB Function : MATLABFcn  MATLABFcn=zerr  OutputDimensions=1
  Interpreted MATLAB Function1 : MATLABFcn  MATLABFcn=zrateerr
  Mux : Mux  Inputs=2
  Mux1 : Mux  Inputs=2
  Scope : Scope
      settings: SaveName=ScopeData25
  Scope1 : Scope
      settings: YMin=-30  YMax=30  SaveName=ScopeData24
  Scope2 : Scope
      settings: SaveName=ScopeData27
  z control : simulink/Continuous/PID Controller  Controller=PID  TimeDomain=Continuous-time  SampleTime=1  IntegratorMethod=Forward Euler  FilterMethod=Forward Euler  Form=Parallel  P=1  I=0  D=0  N=100  InitialConditionSource=internal  InitialConditionForIntegrator=0  InitialConditionForFilter=0  ExternalReset=none  LimitOutput=on  UpperSaturationLimit=2.5  LowerSaturationLimit=-1.6  LinearizeAsGain=off  AntiWindupMode=clamping  Kb=1  TrackingMode=off  Kt=1  PParamMin=[]  PParamMax=[]  IParamMin=[]  IParamMax=[]  DParamMin=[]  DParamMax=[]  NParamMin=[]  NParamMax=[]  KbParamMin=[]  KbParamMax=[]  KtParamMin=[]  KtParamMax=[]  POutMin=[]  POutMax=[]  IOutMin=[]  IOutMax=[]  DOutMin=[]  DOutMax=[]  NOutMin=[]  NOutMax=[]  KbOutMin=[]  KbOutMax=[]  KtOutMin=[]  KtOutMax=[]  IntegratorOutMin=[]  IntegratorOutMax=[]  FilterOutMin=[]  FilterOutMax=[]  SumOutMin=[]  SumOutMax=[]  SumI1OutMin=[]  SumI1OutMax=[]  SumI2OutMin=[]  SumI2OutMax=[]  SumI3OutMin=[]  SumI3OutMax=[]  SumDOutMin=[]  SumDOutMax=[]  SaturationOutMin=[]  SaturationOutMax=[]  IntegratorContinuousStateAttributes=''  IntegratorStateMustResolveToSignalObject=off  IntegratorRTWStateStorageClass=Auto  FilterContinuousStateAttributes=''  FilterStateMustResolveToSignalObject=off  FilterRTWStateStorageClass=Auto
  z rate control : simulink/Continuous/PID Controller  Controller=PID  TimeDomain=Continuous-time  SampleTime=1  IntegratorMethod=Forward Euler  FilterMethod=Forward Euler  Form=Parallel  P=5  I=2  D=4  N=100  InitialConditionSource=internal  InitialConditionForIntegrator=0  InitialConditionForFilter=0  ExternalReset=none  LimitOutput=off  UpperSaturationLimit=2.5  LowerSaturationLimit=-2.5  LinearizeAsGain=off  AntiWindupMode=clamping  Kb=1  TrackingMode=off  Kt=1  PParamMin=[]  PParamMax=[]  IParamMin=[]  IParamMax=[]  DParamMin=[]  DParamMax=[]  NParamMin=[]  NParamMax=[]  KbParamMin=[]  KbParamMax=[]  KtParamMin=[]  KtParamMax=[]  POutMin=[]  POutMax=[]  IOutMin=[]  IOutMax=[]  DOutMin=[]  DOutMax=[]  NOutMin=[]  NOutMax=[]  KbOutMin=[]  KbOutMax=[]  KtOutMin=[]  KtOutMax=[]  IntegratorOutMin=[]  IntegratorOutMax=[]  FilterOutMin=[]  FilterOutMax=[]  SumOutMin=[]  SumOutMax=[]  SumI1OutMin=[]  SumI1OutMax=[]  SumI2OutMin=[]  SumI2OutMax=[]  SumI3OutMin=[]  SumI3OutMax=[]  SumDOutMin=[]  SumDOutMax=[]  SaturationOutMin=[]  SaturationOutMax=[]  IntegratorContinuousStateAttributes=''  IntegratorStateMustResolveToSignalObject=off  IntegratorRTWStateStorageClass=Auto  FilterContinuousStateAttributes=''  FilterStateMustResolveToSignalObject=off  FilterRTWStateStorageClass=Auto
  Out1 : Outport
  wires:
  States/1 -> Mux/1, Mux1/1
  Zd/1 -> Mux/2
  Mux/1 -> Interpreted MATLAB Function/1
  Interpreted MATLAB Function/1 -> z control/1, Scope2/1
  z control/1 -> Scope1/1, Mux1/2
  Mux1/1 -> Interpreted MATLAB Function1/1
  Interpreted MATLAB Function1/1 -> Scope/1, z rate control/1
  z rate control/1 -> Out1/1

== system SystemPIDClosedLoop_motor_closed_zrate_cascade/Motors1/motor1 ==
  DesiredThrust : Inport
  ThrustCoeff : Inport  Port=2  PortDimensions=1
  Interpreted MATLAB Function : MATLABFcn  MATLABFcn=motor1
  Mux : Mux  Inputs=2
  Transfer Fcn : TransferFcn  Numerator=[0 0.936]  Denominator=[0.178 1]
  Actual Omega : Outport
  wires:
  DesiredThrust/1 -> Mux/1
  ThrustCoeff/1 -> Mux/2
  Mux/1 -> Interpreted MATLAB Function/1
  Interpreted MATLAB Function/1 -> Transfer Fcn/1
  Transfer Fcn/1 -> Actual Omega/1

== system SystemPIDClosedLoop_motor_closed_zrate_cascade/Motors1/motor2 ==
  DesiredThrust : Inport
  ThrustCoeff : Inport  Port=2  PortDimensions=1
  Interpreted MATLAB Function : MATLABFcn  MATLABFcn=motor2
  Mux : Mux  Inputs=2
  Transfer Fcn : TransferFcn  Numerator=[0 0.936]  Denominator=[0.178 1]
  Actual Omega : Outport
  wires:
  ThrustCoeff/1 -> Mux/2
  DesiredThrust/1 -> Mux/1
  Mux/1 -> Interpreted MATLAB Function/1
  Interpreted MATLAB Function/1 -> Transfer Fcn/1
  Transfer Fcn/1 -> Actual Omega/1

== system SystemPIDClosedLoop_motor_closed_zrate_cascade/Motors1/motor3 ==
  DesiredThrust : Inport
  ThrustCoeff : Inport  Port=2  PortDimensions=1
  Interpreted MATLAB Function : MATLABFcn  MATLABFcn=motor3
  Mux : Mux  Inputs=2
  Transfer Fcn : TransferFcn  Numerator=[0 0.936]  Denominator=[0.178 1]
  desired omega : Scope
      settings: YMin=0  YMax=350  SaveName=ScopeData29
  Actual Omega : Outport
  wires:
  DesiredThrust/1 -> Mux/1
  ThrustCoeff/1 -> Mux/2
  Mux/1 -> Interpreted MATLAB Function/1
  Interpreted MATLAB Function/1 -> desired omega/1, Transfer Fcn/1
  Transfer Fcn/1 -> Actual Omega/1

== system SystemPIDClosedLoop_motor_closed_zrate_cascade/Motors1/motor4 ==
  DesiredThrust : Inport
  ThrustCoeff : Inport  Port=2  PortDimensions=1
  Mux : Mux  Inputs=2
  Transfer Fcn : TransferFcn  Numerator=[0 0.936]  Denominator=[0.178 1]
  motor4 : MATLABFcn  MATLABFcn=motor4
  Actual Omega : Outport
  wires:
  DesiredThrust/1 -> Mux/1
  ThrustCoeff/1 -> Mux/2
  Mux/1 -> motor4/1
  motor4/1 -> Transfer Fcn/1
  Transfer Fcn/1 -> Actual Omega/1
